simulink model "TST_EISGov_SelectParameter"  (R2016b)
settings: Solver=FixedStepDiscrete  StartTime=0.0  StopTime=simTime  FixedStep=sampleTime  RelTol=1e-3
values from neighbouring files (symbols this model uses):
  testCase = 1    [initTST_EISGov_SelectParameter_001.m]
libraries: simulink x26, UnitTest_Lib x24
(part 1 of 3)
settings Model: Creator=zhengjinyan  LastModifiedBy=zhengjinyan
settings DebuggingCC: SignalRangeChecking=error

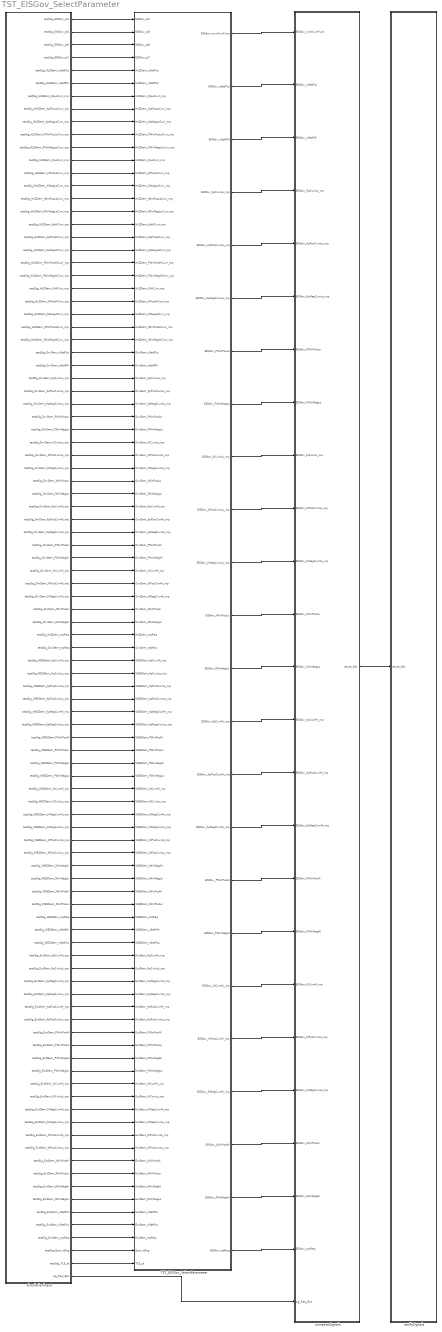
== system TST_EISGov_SelectParameter ==
  TST_EISGov_SelectParameter : Subsystem
  compareSignals : Subsystem
  simulationInput : Subsystem
  verifySignals : Subsystem
  wires:
  simulationInput/1(testSig_EISGov_st1) -> TST_EISGov_SelectParameter/1(EISGov_st1)
  simulationInput/2(testSig_EISGov_st3) -> TST_EISGov_SelectParameter/2(EISGov_st3)
  simulationInput/3(testSig_EISGov_st6) -> TST_EISGov_SelectParameter/3(EISGov_st6)
  simulationInput/4(testSig_EISGov_st7) -> TST_EISGov_SelectParameter/4(EISGov_st7)
  simulationInput/5(testSig_HLSDem_nSetPLo) -> TST_EISGov_SelectParameter/5(HLSDem_nSetPLo)
  simulationInput/6(testSig_HLSDem_nSetPHi) -> TST_EISGov_SelectParameter/6(HLSDem_nSetPHi)
  simulationInput/7(testSig_HLSDem_KpLoCurr_mp) -> TST_EISGov_SelectParameter/7(HLSDem_KpLoCurr_mp)
  simulationInput/8(testSig_HLSDem_KpPosLoCurr_mp) -> TST_EISGov_SelectParameter/8(HLSDem_KpPosLoCurr_mp)
  simulationInput/9(testSig_HLSDem_KpNegLoCurr_mp) -> TST_EISGov_SelectParameter/9(HLSDem_KpNegLoCurr_mp)
  simulationInput/10(testSig_HLSDem_PWinPosLoCurr_mp) -> TST_EISGov_SelectParameter/10(HLSDem_PWinPosLoCurr_mp)
  simulationInput/11(testSig_HLSDem_PWinNegLoCurr_mp) -> TST_EISGov_SelectParameter/11(HLSDem_PWinNegLoCurr_mp)
  simulationInput/12(testSig_HLSDem_KiLoCurr_mp) -> TST_EISGov_SelectParameter/12(HLSDem_KiLoCurr_mp)
  simulationInput/13(testSig_HLSDem_KiPosLoCurr_mp) -> TST_EISGov_SelectParameter/13(HLSDem_KiPosLoCurr_mp)
  simulationInput/14(testSig_HLSDem_KiNegLoCurr_mp) -> TST_EISGov_SelectParameter/14(HLSDem_KiNegLoCurr_mp)
  simulationInput/15(testSig_HLSDem_IWinPosLoCurr_mp) -> TST_EISGov_SelectParameter/15(HLSDem_IWinPosLoCurr_mp)
  simulationInput/16(testSig_HLSDem_IWinNegLoCurr_mp) -> TST_EISGov_SelectParameter/16(HLSDem_IWinNegLoCurr_mp)
  simulationInput/17(testSig_HLSDem_KpHiCurr_mp) -> TST_EISGov_SelectParameter/17(HLSDem_KpHiCurr_mp)
  simulationInput/18(testSig_HLSDem_KpPosHiCurr_mp) -> TST_EISGov_SelectParameter/18(HLSDem_KpPosHiCurr_mp)
  simulationInput/19(testSig_HLSDem_KpNegHiCurr_mp) -> TST_EISGov_SelectParameter/19(HLSDem_KpNegHiCurr_mp)
  simulationInput/20(testSig_HLSDem_PWinPosHiCurr_mp) -> TST_EISGov_SelectParameter/20(HLSDem_PWinPosHiCurr_mp)
  simulationInput/21(testSig_HLSDem_PWinNegHiCurr_mp) -> TST_EISGov_SelectParameter/21(HLSDem_PWinNegHiCurr_mp)
  simulationInput/22(testSig_HLSDem_KiHiCurr_mp) -> TST_EISGov_SelectParameter/22(HLSDem_KiHiCurr_mp)
  simulationInput/23(testSig_HLSDem_KiPosHiCurr_mp) -> TST_EISGov_SelectParameter/23(HLSDem_KiPosHiCurr_mp)
  simulationInput/24(testSig_HLSDem_KiNegHiCurr_mp) -> TST_EISGov_SelectParameter/24(HLSDem_KiNegHiCurr_mp)
  simulationInput/25(testSig_HLSDem_IWinPosHiCurr_mp) -> TST_EISGov_SelectParameter/25(HLSDem_IWinPosHiCurr_mp)
  simulationInput/26(testSig_HLSDem_IWinNegHiCurr_mp) -> TST_EISGov_SelectParameter/26(HLSDem_IWinNegHiCurr_mp)
  simulationInput/27(testSig_DrvDem_nSetPLo) -> TST_EISGov_SelectParameter/27(DrvDem_nSetPLo)
  simulationInput/28(testSig_DrvDem_nSetPHi) -> TST_EISGov_SelectParameter/28(DrvDem_nSetPHi)
  simulationInput/29(testSig_DrvDem_KpCurrLo_mp) -> TST_EISGov_SelectParameter/29(DrvDem_KpCurrLo_mp)
  simulationInput/30(testSig_DrvDem_KpPosCurrLo_mp) -> TST_EISGov_SelectParameter/30(DrvDem_KpPosCurrLo_mp)
  simulationInput/31(testSig_DrvDem_KpNegCurrLo_mp) -> TST_EISGov_SelectParameter/31(DrvDem_KpNegCurrLo_mp)
  simulationInput/32(testSig_DrvDem_PWinPosLo) -> TST_EISGov_SelectParameter/32(DrvDem_PWinPosLo)
  simulationInput/33(testSig_DrvDem_PWinNegLo) -> TST_EISGov_SelectParameter/33(DrvDem_PWinNegLo)
  simulationInput/34(testSig_DrvDem_KiCurrLo_mp) -> TST_EISGov_SelectParameter/34(DrvDem_KiCurrLo_mp)
  simulationInput/35(testSig_DrvDem_KiPosCurrLo_mp) -> TST_EISGov_SelectParameter/35(DrvDem_KiPosCurrLo_mp)
  simulationInput/36(testSig_DrvDem_KiNegCurrLo_mp) -> TST_EISGov_SelectParameter/36(DrvDem_KiNegCurrLo_mp)
  simulationInput/37(testSig_DrvDem_IWinPosLo) -> TST_EISGov_SelectParameter/37(DrvDem_IWinPosLo)
  simulationInput/38(testSig_DrvDem_IWinNegLo) -> TST_EISGov_SelectParameter/38(DrvDem_IWinNegLo)
  simulationInput/39(testSig_DrvDem_KpCurrHi_mp) -> TST_EISGov_SelectParameter/39(DrvDem_KpCurrHi_mp)
  simulationInput/40(testSig_DrvDem_KpPosCurrHi_mp) -> TST_EISGov_SelectParameter/40(DrvDem_KpPosCurrHi_mp)
  simulationInput/41(testSig_DrvDem_KpNegCurrHi_mp) -> TST_EISGov_SelectParameter/41(DrvDem_KpNegCurrHi_mp)
  simulationInput/42(testSig_DrvDem_PWinPosHi) -> TST_EISGov_SelectParameter/42(DrvDem_PWinPosHi)
  simulationInput/43(testSig_DrvDem_PWinNegHi) -> TST_EISGov_SelectParameter/43(DrvDem_PWinNegHi)
  simulationInput/44(testSig_DrvDem_KiCurrHi_mp) -> TST_EISGov_SelectParameter/44(DrvDem_KiCurrHi_mp)
  simulationInput/45(testSig_DrvDem_KiPosCurrHi_mp) -> TST_EISGov_SelectParameter/45(DrvDem_KiPosCurrHi_mp)
  simulationInput/46(testSig_DrvDem_KiNegCurrHi_mp) -> TST_EISGov_SelectParameter/46(DrvDem_KiNegCurrHi_mp)
  simulationInput/47(testSig_DrvDem_IWinPosHi) -> TST_EISGov_SelectParameter/47(DrvDem_IWinPosHi)
  simulationInput/48(testSig_DrvDem_IWinNegHi) -> TST_EISGov_SelectParameter/48(DrvDem_IWinNegHi)
  simulationInput/49(testSig_HLSDem_trqReq) -> TST_EISGov_SelectParameter/49(HLSDem_trqReq)
  simulationInput/50(testSig_DrvDem_trqReq) -> TST_EISGov_SelectParameter/50(DrvDem_trqReq)
  simulationInput/51(testSig_WESDem_KpCurrHi_mp) -> TST_EISGov_SelectParameter/51(WESDem_KpCurrHi_mp)
  simulationInput/52(testSig_WESDem_KpCurrLo_mp) -> TST_EISGov_SelectParameter/52(WESDem_KpCurrLo_mp)
  simulationInput/53(testSig_WESDem_KpPosCurrHi_mp) -> TST_EISGov_SelectParameter/53(WESDem_KpPosCurrHi_mp)
  simulationInput/54(testSig_WESDem_KpPosCurrLo_mp) -> TST_EISGov_SelectParameter/54(WESDem_KpPosCurrLo_mp)
  simulationInput/55(testSig_WESDem_KpNegCurrHi_mp) -> TST_EISGov_SelectParameter/55(WESDem_KpNegCurrHi_mp)
  simulationInput/56(testSig_WESDem_KpNegCurrLo_mp) -> TST_EISGov_SelectParameter/56(WESDem_KpNegCurrLo_mp)
  simulationInput/57(testSig_WESDem_PWinPosHi) -> TST_EISGov_SelectParameter/57(WESDem_PWinPosHi)
  simulationInput/58(testSig_WESDem_PWinPosLo) -> TST_EISGov_SelectParameter/58(WESDem_PWinPosLo)
  simulationInput/59(testSig_WESDem_PWinNegHi) -> TST_EISGov_SelectParameter/59(WESDem_PWinNegHi)
  simulationInput/60(testSig_WESDem_PWinNegLo) -> TST_EISGov_SelectParameter/60(WESDem_PWinNegLo)
  simulationInput/61(testSig_WESDem_KiCurrHi_mp) -> TST_EISGov_SelectParameter/61(WESDem_KiCurrHi_mp)
  simulationInput/62(testSig_WESDem_KiCurrLo_mp) -> TST_EISGov_SelectParameter/62(WESDem_KiCurrLo_mp)
  simulationInput/63(testSig_WESDem_KiNegCurrHi_mp) -> TST_EISGov_SelectParameter/63(WESDem_KiNegCurrHi_mp)
  simulationInput/64(testSig_WESDem_KiNegCurrLo_mp) -> TST_EISGov_SelectParameter/64(WESDem_KiNegCurrLo_mp)
  simulationInput/65(testSig_WESDem_KiPosCurrHi_mp) -> TST_EISGov_SelectParameter/65(WESDem_KiPosCurrHi_mp)
  simulationInput/66(testSig_WESDem_KiPosCurrLo_mp) -> TST_EISGov_SelectParameter/66(WESDem_KiPosCurrLo_mp)
  simulationInput/67(testSig_WESDem_IWinNegHi) -> TST_EISGov_SelectParameter/67(WESDem_IWinNegHi)
  simulationInput/68(testSig_WESDem_IWinNegLo) -> TST_EISGov_SelectParameter/68(WESDem_IWinNegLo)
  simulationInput/69(testSig_WESDem_IWinPosHi) -> TST_EISGov_SelectParameter/69(WESDem_IWinPosHi)
  simulationInput/70(testSig_WESDem_IWinPosLo) -> TST_EISGov_SelectParameter/70(WESDem_IWinPosLo)
  simulationInput/71(testSig_WESDem_trqReq) -> TST_EISGov_SelectParameter/71(WESDem_trqReq)
  simulationInput/72(testSig_WESDem_nSetPHi) -> TST_EISGov_SelectParameter/72(WESDem_nSetPHi)
  simulationInput/73(testSig_WESDem_nSetPLo) -> TST_EISGov_SelectParameter/73(WESDem_nSetPLo)
  simulationInput/74(testSig_ExtDem_KpCurrHi_mp) -> TST_EISGov_SelectParameter/74(ExtDem_KpCurrHi_mp)
  simulationInput/75(testSig_ExtDem_KpCurrLo_mp) -> TST_EISGov_SelectParameter/75(ExtDem_KpCurrLo_mp)
  simulationInput/76(testSig_ExtDem_KpNegCurrHi_mp) -> TST_EISGov_SelectParameter/76(ExtDem_KpNegCurrHi_mp)
  simulationInput/77(testSig_ExtDem_KpNegCurrLo_mp) -> TST_EISGov_SelectParameter/77(ExtDem_KpNegCurrLo_mp)
  simulationInput/78(testSig_ExtDem_KpPosCurrHi_mp) -> TST_EISGov_SelectParameter/78(ExtDem_KpPosCurrHi_mp)
  simulationInput/79(testSig_ExtDem_KpPosCurrLo_mp) -> TST_EISGov_SelectParameter/79(ExtDem_KpPosCurrLo_mp)
  simulationInput/80(testSig_ExtDem_PWinPosHi) -> TST_EISGov_SelectParameter/80(ExtDem_PWinPosHi)
  simulationInput/81(testSig_ExtDem_PWinPosLo) -> TST_EISGov_SelectParameter/81(ExtDem_PWinPosLo)
  simulationInput/82(testSig_ExtDem_PWinNegHi) -> TST_EISGov_SelectParameter/82(ExtDem_PWinNegHi)
  simulationInput/83(testSig_ExtDem_PWinNegLo) -> TST_EISGov_SelectParameter/83(ExtDem_PWinNegLo)
  simulationInput/84(testSig_ExtDem_KiCurrHi_mp) -> TST_EISGov_SelectParameter/84(ExtDem_KiCurrHi_mp)
  simulationInput/85(testSig_ExtDem_KiCurrLo_mp) -> TST_EISGov_SelectParameter/85(ExtDem_KiCurrLo_mp)
  simulationInput/86(testSig_ExtDem_KiNegCurrHi_mp) -> TST_EISGov_SelectParameter/86(ExtDem_KiNegCurrHi_mp)
  simulationInput/87(testSig_ExtDem_KiNegCurrLo_mp) -> TST_EISGov_SelectParameter/87(ExtDem_KiNegCurrLo_mp)
  simulationInput/88(testSig_ExtDem_KiPosCurrHi_mp) -> TST_EISGov_SelectParameter/88(ExtDem_KiPosCurrHi_mp)
  simulationInput/89(testSig_ExtDem_KiPosCurrLo_mp) -> TST_EISGov_SelectParameter/89(ExtDem_KiPosCurrLo_mp)
  simulationInput/90(testSig_ExtDem_IWinPosHi) -> TST_EISGov_SelectParameter/90(ExtDem_IWinPosHi)
  simulationInput/91(testSig_ExtDem_IWinPosLo) -> TST_EISGov_SelectParameter/91(ExtDem_IWinPosLo)
  simulationInput/92(testSig_ExtDem_IWinNegHi) -> TST_EISGov_SelectParameter/92(ExtDem_IWinNegHi)
  simulationInput/93(testSig_ExtDem_IWinNegLo) -> TST_EISGov_SelectParameter/93(ExtDem_IWinNegLo)
  simulationInput/94(testSig_ExtDem_nSetPHi) -> TST_EISGov_SelectParameter/94(ExtDem_nSetPHi)
  simulationInput/95(testSig_ExtDem_nSetPLo) -> TST_EISGov_SelectParameter/95(ExtDem_nSetPLo)
  simulationInput/96(testSig_ExtDem_trqReq) -> TST_EISGov_SelectParameter/96(ExtDem_trqReq)
  simulationInput/97(testSig_Epm_nEng) -> TST_EISGov_SelectParameter/97(Epm_nEng)
  simulationInput/98(testSig_T15_st) -> TST_EISGov_SelectParameter/98(T15_st)
  TST_EISGov_SelectParameter/1(EISGov_numCurrFunc) -> compareSignals/1(EISGov_numCurrFunc)
  TST_EISGov_SelectParameter/2(EISGov_nSetPLo) -> compareSignals/2(EISGov_nSetPLo)
  TST_EISGov_SelectParameter/3(EISGov_nSetPHi) -> compareSignals/3(EISGov_nSetPHi)
  TST_EISGov_SelectParameter/4(EISGov_KpCurrLo_mp) -> compareSignals/4(EISGov_KpCurrLo_mp)
  TST_EISGov_SelectParameter/5(EISGov_KpPosCurrLo_mp) -> compareSignals/5(EISGov_KpPosCurrLo_mp)
  TST_EISGov_SelectParameter/6(EISGov_KpNegCurrLo_mp) -> compareSignals/6(EISGov_KpNegCurrLo_mp)
  TST_EISGov_SelectParameter/7(EISGov_PWinPosLo) -> compareSignals/7(EISGov_PWinPosLo)
  TST_EISGov_SelectParameter/8(EISGov_PWinNegLo) -> compareSignals/8(EISGov_PWinNegLo)
  TST_EISGov_SelectParameter/9(EISGov_KiCurrLo_mp) -> compareSignals/9(EISGov_KiCurrLo_mp)
  TST_EISGov_SelectParameter/10(EISGov_KiPosCurrLo_mp) -> compareSignals/10(EISGov_KiPosCurrLo_mp)
  TST_EISGov_SelectParameter/11(EISGov_KiNegCurrLo_mp) -> compareSignals/11(EISGov_KiNegCurrLo_mp)
  TST_EISGov_SelectParameter/12(EISGov_IWinPosLo) -> compareSignals/12(EISGov_IWinPosLo)
  TST_EISGov_SelectParameter/13(EISGov_IWinNegLo) -> compareSignals/13(EISGov_IWinNegLo)
  TST_EISGov_SelectParameter/14(EISGov_KpCurrHi_mp) -> compareSignals/14(EISGov_KpCurrHi_mp)
  TST_EISGov_SelectParameter/15(EISGov_KpPosCurrHi_mp) -> compareSignals/15(EISGov_KpPosCurrHi_mp)
  TST_EISGov_SelectParameter/16(EISGov_KpNegCurrHi_mp) -> compareSignals/16(EISGov_KpNegCurrHi_mp)
  TST_EISGov_SelectParameter/17(EISGov_PWinPosHi) -> compareSignals/17(EISGov_PWinPosHi)
  TST_EISGov_SelectParameter/18(EISGov_PWinNegHi) -> compareSignals/18(EISGov_PWinNegHi)
  TST_EISGov_SelectParameter/19(EISGov_KiCurrHi_mp) -> compareSignals/19(EISGov_KiCurrHi_mp)
  TST_EISGov_SelectParameter/20(EISGov_KiPosCurrHi_mp) -> compareSignals/20(EISGov_KiPosCurrHi_mp)
  TST_EISGov_SelectParameter/21(EISGov_KiNegCurrHi_mp) -> compareSignals/21(EISGov_KiNegCurrHi_mp)
  TST_EISGov_SelectParameter/22(EISGov_IWinPosHi) -> compareSignals/22(EISGov_IWinPosHi)
  TST_EISGov_SelectParameter/23(EISGov_IWinNegHi) -> compareSignals/23(EISGov_IWinNegHi)
  TST_EISGov_SelectParameter/24(EISGov_trqReq) -> compareSignals/24(EISGov_trqReq)
  simulationInput/99(sig_Req_Bus) -> compareSignals/25(sig_Req_Bus)
  compareSignals/1(result_001) -> verifySignals/1(result_001)

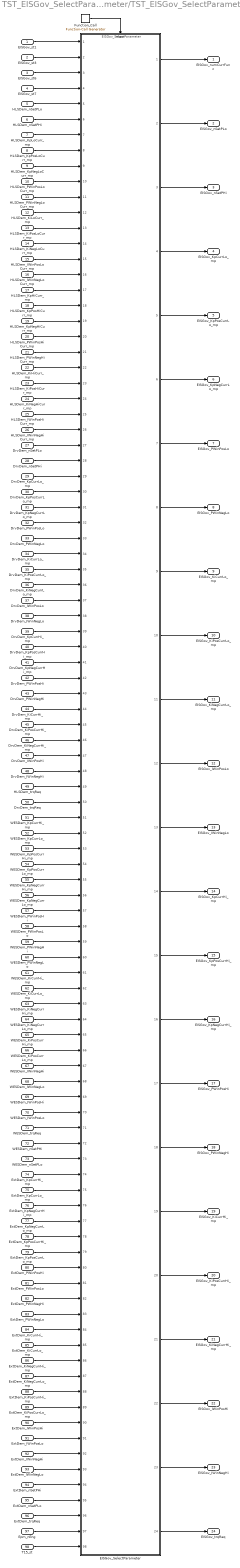
== system TST_EISGov_SelectParameter/TST_EISGov_SelectParameter ==
  EISGov_st1 : Inport
  EISGov_st3 : Inport  Port=2
  EISGov_st6 : Inport  Port=3
  EISGov_st7 : Inport  Port=4
  HLSDem_nSetPLo : Inport  Port=5
  HLSDem_nSetPHi : Inport  Port=6
  HLSDem_KpLoCurr_mp : Inport  Port=7
  HLSDem_KpPosLoCurr_mp : Inport  Port=8
  HLSDem_KpNegLoCurr_mp : Inport  Port=9
  HLSDem_PWinPosLoCurr_mp : Inport  Port=10
  HLSDem_PWinNegLoCurr_mp : Inport  Port=11
  HLSDem_KiLoCurr_mp : Inport  Port=12
  HLSDem_KiPosLoCurr_mp : Inport  Port=13
  HLSDem_KiNegLoCurr_mp : Inport  Port=14
  HLSDem_IWinPosLoCurr_mp : Inport  Port=15
  HLSDem_IWinNegLoCurr_mp : Inport  Port=16
  HLSDem_KpHiCurr_mp : Inport  Port=17
  HLSDem_KpPosHiCurr_mp : Inport  Port=18
  HLSDem_KpNegHiCurr_mp : Inport  Port=19
  HLSDem_PWinPosHiCurr_mp : Inport  Port=20
  HLSDem_PWinNegHiCurr_mp : Inport  Port=21
  HLSDem_KiHiCurr_mp : Inport  Port=22
  HLSDem_KiPosHiCurr_mp : Inport  Port=23
  HLSDem_KiNegHiCurr_mp : Inport  Port=24
  HLSDem_IWinPosHiCurr_mp : Inport  Port=25
  HLSDem_IWinNegHiCurr_mp : Inport  Port=26
  DrvDem_nSetPLo : Inport  Port=27
  DrvDem_nSetPHi : Inport  Port=28
  DrvDem_KpCurrLo_mp : Inport  Port=29
  DrvDem_KpPosCurrLo_mp : Inport  Port=30
  DrvDem_KpNegCurrLo_mp : Inport  Port=31
  DrvDem_PWinPosLo : Inport  Port=32
  DrvDem_PWinNegLo : Inport  Port=33
  DrvDem_KiCurrLo_mp : Inport  Port=34
  DrvDem_KiPosCurrLo_mp : Inport  Port=35
  DrvDem_KiNegCurrLo_mp : Inport  Port=36
  DrvDem_IWinPosLo : Inport  Port=37
  DrvDem_IWinNegLo : Inport  Port=38
  DrvDem_KpCurrHi_mp : Inport  Port=39
  DrvDem_KpPosCurrHi_mp : Inport  Port=40
  DrvDem_KpNegCurrHi_mp : Inport  Port=41
  DrvDem_PWinPosHi : Inport  Port=42
  DrvDem_PWinNegHi : Inport  Port=43
  DrvDem_KiCurrHi_mp : Inport  Port=44
  DrvDem_KiPosCurrHi_mp : Inport  Port=45
  DrvDem_KiNegCurrHi_mp : Inport  Port=46
  DrvDem_IWinPosHi : Inport  Port=47
  DrvDem_IWinNegHi : Inport  Port=48
  HLSDem_trqReq : Inport  Port=49
  DrvDem_trqReq : Inport  Port=50
  WESDem_KpCurrHi_mp : Inport  Port=51
  WESDem_KpCurrLo_mp : Inport  Port=52
  WESDem_KpPosCurrHi_mp : Inport  Port=53
  WESDem_KpPosCurrLo_mp : Inport  Port=54
  WESDem_KpNegCurrHi_mp : Inport  Port=55
  WESDem_KpNegCurrLo_mp : Inport  Port=56
  WESDem_PWinPosHi : Inport  Port=57
  WESDem_PWinPosLo : Inport  Port=58
  WESDem_PWinNegHi : Inport  Port=59
  WESDem_PWinNegLo : Inport  Port=60
  WESDem_KiCurrHi_mp : Inport  Port=61
  WESDem_KiCurrLo_mp : Inport  Port=62
  WESDem_KiNegCurrHi_mp : Inport  Port=63
  WESDem_KiNegCurrLo_mp : Inport  Port=64
  WESDem_KiPosCurrHi_mp : Inport  Port=65
  WESDem_KiPosCurrLo_mp : Inport  Port=66
  WESDem_IWinNegHi : Inport  Port=67
  WESDem_IWinNegLo : Inport  Port=68
  WESDem_IWinPosHi : Inport  Port=69
  WESDem_IWinPosLo : Inport  Port=70
  WESDem_trqReq : Inport  Port=71
  WESDem_nSetPHi : Inport  Port=72
  WESDem_nSetPLo : Inport  Port=73
  ExtDem_KpCurrHi_mp : Inport  Port=74
  ExtDem_KpCurrLo_mp : Inport  Port=75
  ExtDem_KpNegCurrHi_mp : Inport  Port=76
  ExtDem_KpNegCurrLo_mp : Inport  Port=77
  ExtDem_KpPosCurrHi_mp : Inport  Port=78
  ExtDem_KpPosCurrLo_mp : Inport  Port=79
  ExtDem_PWinPosHi : Inport  Port=80
  ExtDem_PWinPosLo : Inport  Port=81
  ExtDem_PWinNegHi : Inport  Port=82
  ExtDem_PWinNegLo : Inport  Port=83
  ExtDem_KiCurrHi_mp : Inport  Port=84
  ExtDem_KiCurrLo_mp : Inport  Port=85
  ExtDem_KiNegCurrHi_mp : Inport  Port=86
  ExtDem_KiNegCurrLo_mp : Inport  Port=87
  ExtDem_KiPosCurrHi_mp : Inport  Port=88
  ExtDem_KiPosCurrLo_mp : Inport  Port=89
  ExtDem_IWinPosHi : Inport  Port=90
  ExtDem_IWinPosLo : Inport  Port=91
  ExtDem_IWinNegHi : Inport  Port=92
  ExtDem_IWinNegLo : Inport  Port=93
  ExtDem_nSetPHi : Inport  Port=94
  ExtDem_nSetPLo : Inport  Port=95
  ExtDem_trqReq : Inport  Port=96
  Epm_nEng : Inport  Port=97
  T15_st : Inport  Port=98
  EISGov_SelectParameter : ModelReference  ModelNameDialog=EISGov_SelectParameter  SimulationMode=Normal  ModelReferenceVersion=1.180  TriggerPortName=function  TriggerPortTriggerType=function-call  TriggerPortStatesWhenEnabling=held
  Function_Call : simulink/Ports & Subsystems/Function-Call Generator  sample_time=sampleTime  numberOfIterations=1
  EISGov_numCurrFunc : Outport
  EISGov_nSetPLo : Outport  Port=2
  EISGov_nSetPHi : Outport  Port=3
  EISGov_KpCurrLo_mp : Outport  Port=4
  EISGov_KpPosCurrLo_mp : Outport  Port=5
  EISGov_KpNegCurrLo_mp : Outport  Port=6
  EISGov_PWinPosLo : Outport  Port=7
  EISGov_PWinNegLo : Outport  Port=8
  EISGov_KiCurrLo_mp : Outport  Port=9
  EISGov_KiPosCurrLo_mp : Outport  Port=10
  EISGov_KiNegCurrLo_mp : Outport  Port=11
  EISGov_IWinPosLo : Outport  Port=12
  EISGov_IWinNegLo : Outport  Port=13
  EISGov_KpCurrHi_mp : Outport  Port=14
  EISGov_KpPosCurrHi_mp : Outport  Port=15
  EISGov_KpNegCurrHi_mp : Outport  Port=16
  EISGov_PWinPosHi : Outport  Port=17
  EISGov_PWinNegHi : Outport  Port=18
  EISGov_KiCurrHi_mp : Outport  Port=19
  EISGov_KiPosCurrHi_mp : Outport  Port=20
  EISGov_KiNegCurrHi_mp : Outport  Port=21
  EISGov_IWinPosHi : Outport  Port=22
  EISGov_IWinNegHi : Outport  Port=23
  EISGov_trqReq : Outport  Port=24
  wires:
  Function_Call/1 -> EISGov_SelectParameter/Trigger
  EISGov_st1/1 -> EISGov_SelectParameter/1
  EISGov_st3/1 -> EISGov_SelectParameter/2
  EISGov_st6/1 -> EISGov_SelectParameter/3
  EISGov_st7/1 -> EISGov_SelectParameter/4
  HLSDem_nSetPLo/1 -> EISGov_SelectParameter/5
  HLSDem_nSetPHi/1 -> EISGov_SelectParameter/6
  HLSDem_KpLoCurr_mp/1 -> EISGov_SelectParameter/7
  HLSDem_KpPosLoCurr_mp/1 -> EISGov_SelectParameter/8
  HLSDem_KpNegLoCurr_mp/1 -> EISGov_SelectParameter/9
  HLSDem_PWinPosLoCurr_mp/1 -> EISGov_SelectParameter/10
  HLSDem_PWinNegLoCurr_mp/1 -> EISGov_SelectParameter/11
  HLSDem_KiLoCurr_mp/1 -> EISGov_SelectParameter/12
  HLSDem_KiPosLoCurr_mp/1 -> EISGov_SelectParameter/13
  HLSDem_KiNegLoCurr_mp/1 -> EISGov_SelectParameter/14
  HLSDem_IWinPosLoCurr_mp/1 -> EISGov_SelectParameter/15
  HLSDem_IWinNegLoCurr_mp/1 -> EISGov_SelectParameter/16
  HLSDem_KpHiCurr_mp/1 -> EISGov_SelectParameter/17
  HLSDem_KpPosHiCurr_mp/1 -> EISGov_SelectParameter/18
  HLSDem_KpNegHiCurr_mp/1 -> EISGov_SelectParameter/19
  HLSDem_PWinPosHiCurr_mp/1 -> EISGov_SelectParameter/20
  HLSDem_PWinNegHiCurr_mp/1 -> EISGov_SelectParameter/21
  HLSDem_KiHiCurr_mp/1 -> EISGov_SelectParameter/22
  HLSDem_KiPosHiCurr_mp/1 -> EISGov_SelectParameter/23
  HLSDem_KiNegHiCurr_mp/1 -> EISGov_SelectParameter/24
  HLSDem_IWinPosHiCurr_mp/1 -> EISGov_SelectParameter/25
  HLSDem_IWinNegHiCurr_mp/1 -> EISGov_SelectParameter/26
  DrvDem_nSetPLo/1 -> EISGov_SelectParameter/27
  DrvDem_nSetPHi/1 -> EISGov_SelectParameter/28
  DrvDem_KpCurrLo_mp/1 -> EISGov_SelectParameter/29
  DrvDem_KpPosCurrLo_mp/1 -> EISGov_SelectParameter/30
  DrvDem_KpNegCurrLo_mp/1 -> EISGov_SelectParameter/31
  DrvDem_PWinPosLo/1 -> EISGov_SelectParameter/32
  DrvDem_PWinNegLo/1 -> EISGov_SelectParameter/33
  DrvDem_KiCurrLo_mp/1 -> EISGov_SelectParameter/34
  DrvDem_KiPosCurrLo_mp/1 -> EISGov_SelectParameter/35
  DrvDem_KiNegCurrLo_mp/1 -> EISGov_SelectParameter/36
  DrvDem_IWinPosLo/1 -> EISGov_SelectParameter/37
  DrvDem_IWinNegLo/1 -> EISGov_SelectParameter/38
  DrvDem_KpCurrHi_mp/1 -> EISGov_SelectParameter/39
  DrvDem_KpPosCurrHi_mp/1 -> EISGov_SelectParameter/40
  DrvDem_KpNegCurrHi_mp/1 -> EISGov_SelectParameter/41
  DrvDem_PWinPosHi/1 -> EISGov_SelectParameter/42
  DrvDem_PWinNegHi/1 -> EISGov_SelectParameter/43
  DrvDem_KiCurrHi_mp/1 -> EISGov_SelectParameter/44
  DrvDem_KiPosCurrHi_mp/1 -> EISGov_SelectParameter/45
  DrvDem_KiNegCurrHi_mp/1 -> EISGov_SelectParameter/46
  DrvDem_IWinPosHi/1 -> EISGov_SelectParameter/47
  DrvDem_IWinNegHi/1 -> EISGov_SelectParameter/48
  HLSDem_trqReq/1 -> EISGov_SelectParameter/49
  DrvDem_trqReq/1 -> EISGov_SelectParameter/50
  WESDem_KpCurrHi_mp/1 -> EISGov_SelectParameter/51
  WESDem_KpCurrLo_mp/1 -> EISGov_SelectParameter/52
  WESDem_KpPosCurrHi_mp/1 -> EISGov_SelectParameter/53
  WESDem_KpPosCurrLo_mp/1 -> EISGov_SelectParameter/54
  WESDem_KpNegCurrHi_mp/1 -> EISGov_SelectParameter/55
  WESDem_KpNegCurrLo_mp/1 -> EISGov_SelectParameter/56
  WESDem_PWinPosHi/1 -> EISGov_SelectParameter/57
  WESDem_PWinPosLo/1 -> EISGov_SelectParameter/58
  WESDem_PWinNegHi/1 -> EISGov_SelectParameter/59
  WESDem_PWinNegLo/1 -> EISGov_SelectParameter/60
  WESDem_KiCurrHi_mp/1 -> EISGov_SelectParameter/61
  WESDem_KiCurrLo_mp/1 -> EISGov_SelectParameter/62
  WESDem_KiNegCurrHi_mp/1 -> EISGov_SelectParameter/63
  WESDem_KiNegCurrLo_mp/1 -> EISGov_SelectParameter/64
  WESDem_KiPosCurrHi_mp/1 -> EISGov_SelectParameter/65
  WESDem_KiPosCurrLo_mp/1 -> EISGov_SelectParameter/66
  WESDem_IWinNegHi/1 -> EISGov_SelectParameter/67
  WESDem_IWinNegLo/1 -> EISGov_SelectParameter/68
  WESDem_IWinPosHi/1 -> EISGov_SelectParameter/69
  WESDem_IWinPosLo/1 -> EISGov_SelectParameter/70
  WESDem_trqReq/1 -> EISGov_SelectParameter/71
  WESDem_nSetPHi/1 -> EISGov_SelectParameter/72
  WESDem_nSetPLo/1 -> EISGov_SelectParameter/73
  ExtDem_KpCurrHi_mp/1 -> EISGov_SelectParameter/74
  ExtDem_KpCurrLo_mp/1 -> EISGov_SelectParameter/75
  ExtDem_KpNegCurrHi_mp/1 -> EISGov_SelectParameter/76
  ExtDem_KpNegCurrLo_mp/1 -> EISGov_SelectParameter/77
  ExtDem_KpPosCurrHi_mp/1 -> EISGov_SelectParameter/78
  ExtDem_KpPosCurrLo_mp/1 -> EISGov_SelectParameter/79
  ExtDem_PWinPosHi/1 -> EISGov_SelectParameter/80
  ExtDem_PWinPosLo/1 -> EISGov_SelectParameter/81
  ExtDem_PWinNegHi/1 -> EISGov_SelectParameter/82
  ExtDem_PWinNegLo/1 -> EISGov_SelectParameter/83
  ExtDem_KiCurrHi_mp/1 -> EISGov_SelectParameter/84
  ExtDem_KiCurrLo_mp/1 -> EISGov_SelectParameter/85
  ExtDem_KiNegCurrHi_mp/1 -> EISGov_SelectParameter/86
  ExtDem_KiNegCurrLo_mp/1 -> EISGov_SelectParameter/87
  ExtDem_KiPosCurrHi_mp/1 -> EISGov_SelectParameter/88
  ExtDem_KiPosCurrLo_mp/1 -> EISGov_SelectParameter/89
  ExtDem_IWinPosHi/1 -> EISGov_SelectParameter/90
  ExtDem_IWinPosLo/1 -> EISGov_SelectParameter/91
  ExtDem_IWinNegHi/1 -> EISGov_SelectParameter/92
  ExtDem_IWinNegLo/1 -> EISGov_SelectParameter/93
  ExtDem_nSetPHi/1 -> EISGov_SelectParameter/94
  ExtDem_nSetPLo/1 -> EISGov_SelectParameter/95
  ExtDem_trqReq/1 -> EISGov_SelectParameter/96
  Epm_nEng/1 -> EISGov_SelectParameter/97
  T15_st/1 -> EISGov_SelectParameter/98
  EISGov_SelectParameter/1 -> EISGov_numCurrFunc/1
  EISGov_SelectParameter/2 -> EISGov_nSetPLo/1
  EISGov_SelectParameter/3 -> EISGov_nSetPHi/1
  EISGov_SelectParameter/4 -> EISGov_KpCurrLo_mp/1
  EISGov_SelectParameter/5 -> EISGov_KpPosCurrLo_mp/1
  EISGov_SelectParameter/6 -> EISGov_KpNegCurrLo_mp/1
  EISGov_SelectParameter/7 -> EISGov_PWinPosLo/1
  EISGov_SelectParameter/8 -> EISGov_PWinNegLo/1
  EISGov_SelectParameter/9 -> EISGov_KiCurrLo_mp/1
  EISGov_SelectParameter/10 -> EISGov_KiPosCurrLo_mp/1
  EISGov_SelectParameter/11 -> EISGov_KiNegCurrLo_mp/1
  EISGov_SelectParameter/12 -> EISGov_IWinPosLo/1
  EISGov_SelectParameter/13 -> EISGov_IWinNegLo/1
  EISGov_SelectParameter/14 -> EISGov_KpCurrHi_mp/1
  EISGov_SelectParameter/15 -> EISGov_KpPosCurrHi_mp/1
  EISGov_SelectParameter/16 -> EISGov_KpNegCurrHi_mp/1
  EISGov_SelectParameter/17 -> EISGov_PWinPosHi/1
  EISGov_SelectParameter/18 -> EISGov_PWinNegHi/1
  EISGov_SelectParameter/19 -> EISGov_KiCurrHi_mp/1
  EISGov_SelectParameter/20 -> EISGov_KiPosCurrHi_mp/1
  EISGov_SelectParameter/21 -> EISGov_KiNegCurrHi_mp/1
  EISGov_SelectParameter/22 -> EISGov_IWinPosHi/1
  EISGov_SelectParameter/23 -> EISGov_IWinNegHi/1
  EISGov_SelectParameter/24 -> EISGov_trqReq/1

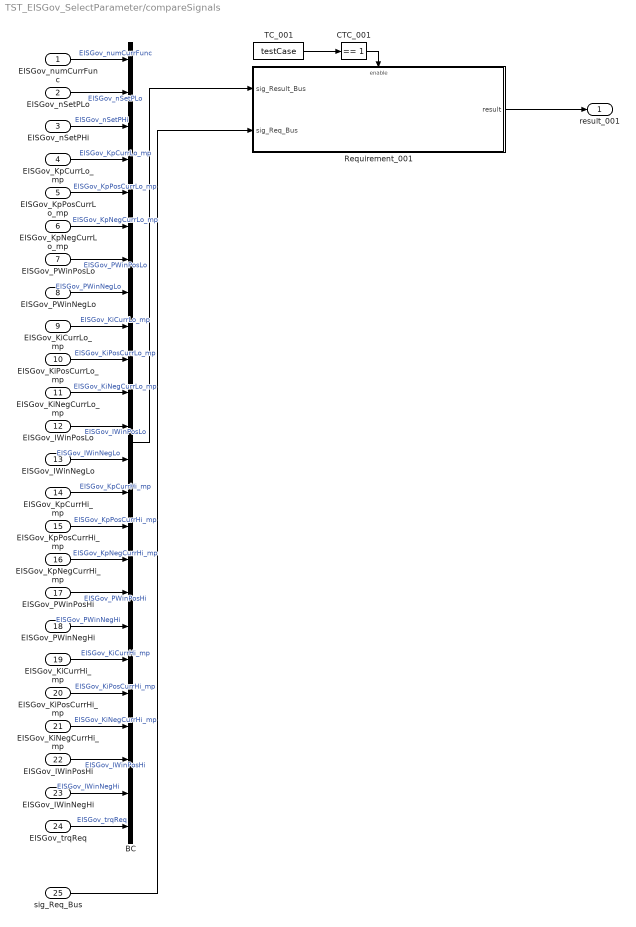
== system TST_EISGov_SelectParameter/compareSignals ==
  EISGov_numCurrFunc : Inport
  EISGov_nSetPLo : Inport  Port=2
  EISGov_nSetPHi : Inport  Port=3
  EISGov_KpCurrLo_mp : Inport  Port=4
  EISGov_KpPosCurrLo_mp : Inport  Port=5
  EISGov_KpNegCurrLo_mp : Inport  Port=6
  EISGov_PWinPosLo : Inport  Port=7
  EISGov_PWinNegLo : Inport  Port=8
  EISGov_KiCurrLo_mp : Inport  Port=9
  EISGov_KiPosCurrLo_mp : Inport  Port=10
  EISGov_KiNegCurrLo_mp : Inport  Port=11
  EISGov_IWinPosLo : Inport  Port=12
  EISGov_IWinNegLo : Inport  Port=13
  EISGov_KpCurrHi_mp : Inport  Port=14
  EISGov_KpPosCurrHi_mp : Inport  Port=15
  EISGov_KpNegCurrHi_mp : Inport  Port=16
  EISGov_PWinPosHi : Inport  Port=17
  EISGov_PWinNegHi : Inport  Port=18
  EISGov_KiCurrHi_mp : Inport  Port=19
  EISGov_KiPosCurrHi_mp : Inport  Port=20
  EISGov_KiNegCurrHi_mp : Inport  Port=21
  EISGov_IWinPosHi : Inport  Port=22
  EISGov_IWinNegHi : Inport  Port=23
  EISGov_trqReq : Inport  Port=24
  sig_Req_Bus : Inport  Port=25
  BC : BusCreator  Inputs=24
  CTC_001 : simulink/Logic and Bit Operations/Compare To Constant  relop===  const=1  OutDataTypeStr=boolean
  Requirement_001 : Subsystem
  TC_001 : Constant  Value=testCase
  result_001 : Outport
  wires:
  EISGov_numCurrFunc/1 -> BC/1  "EISGov_numCurrFunc"
  EISGov_nSetPLo/1 -> BC/2  "EISGov_nSetPLo"
  EISGov_nSetPHi/1 -> BC/3  "EISGov_nSetPHi"
  EISGov_KpCurrLo_mp/1 -> BC/4  "EISGov_KpCurrLo_mp"
  EISGov_KpPosCurrLo_mp/1 -> BC/5  "EISGov_KpPosCurrLo_mp"
  EISGov_KpNegCurrLo_mp/1 -> BC/6  "EISGov_KpNegCurrLo_mp"
  EISGov_PWinPosLo/1 -> BC/7  "EISGov_PWinPosLo"
  EISGov_PWinNegLo/1 -> BC/8  "EISGov_PWinNegLo"
  EISGov_KiCurrLo_mp/1 -> BC/9  "EISGov_KiCurrLo_mp"
  EISGov_KiPosCurrLo_mp/1 -> BC/10  "EISGov_KiPosCurrLo_mp"
  EISGov_KiNegCurrLo_mp/1 -> BC/11  "EISGov_KiNegCurrLo_mp"
  EISGov_IWinPosLo/1 -> BC/12  "EISGov_IWinPosLo"
  EISGov_IWinNegLo/1 -> BC/13  "EISGov_IWinNegLo"
  EISGov_KpCurrHi_mp/1 -> BC/14  "EISGov_KpCurrHi_mp"
  EISGov_KpPosCurrHi_mp/1 -> BC/15  "EISGov_KpPosCurrHi_mp"
  EISGov_KpNegCurrHi_mp/1 -> BC/16  "EISGov_KpNegCurrHi_mp"
  EISGov_PWinPosHi/1 -> BC/17  "EISGov_PWinPosHi"
  EISGov_PWinNegHi/1 -> BC/18  "EISGov_PWinNegHi"
  EISGov_KiCurrHi_mp/1 -> BC/19  "EISGov_KiCurrHi_mp"
  EISGov_KiPosCurrHi_mp/1 -> BC/20  "EISGov_KiPosCurrHi_mp"
  EISGov_KiNegCurrHi_mp/1 -> BC/21  "EISGov_KiNegCurrHi_mp"
  EISGov_IWinPosHi/1 -> BC/22  "EISGov_IWinPosHi"
  EISGov_IWinNegHi/1 -> BC/23  "EISGov_IWinNegHi"
  EISGov_trqReq/1 -> BC/24  "EISGov_trqReq"
  TC_001/1 -> CTC_001/1
  CTC_001/1 -> Requirement_001/Enable
  sig_Req_Bus/1 -> Requirement_001/2(sig_Req_Bus)
  BC/1 -> Requirement_001/1(sig_Result_Bus)
  Requirement_001/1(result) -> result_001/1

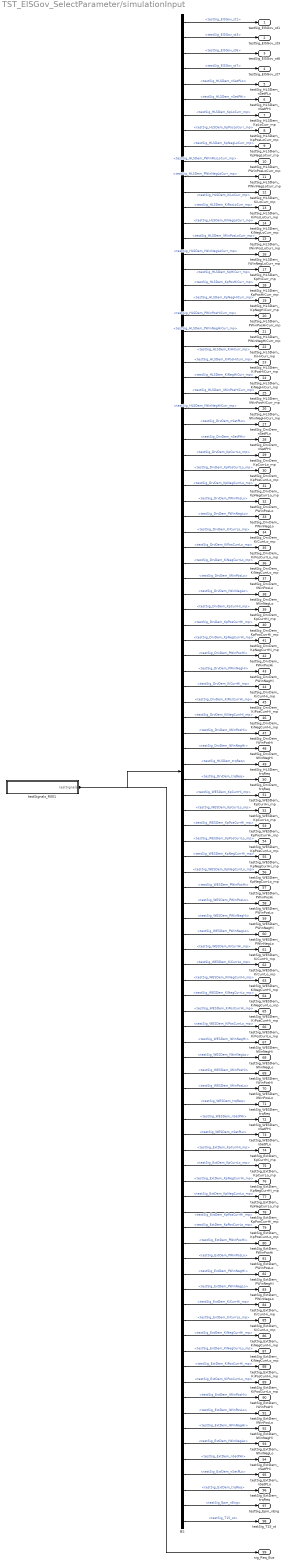
== system TST_EISGov_SelectParameter/simulationInput ==
  BS : BusSelector  OutputSignals=testSig_EISGov_st1,testSig_EISGov_st3,testSig_EISGov_st6,testSig_EISGov_st7,testSig_HLSDem_nSetPLo,testSig_HLSDem_nSetPHi,testSig_HLSDem_KpLoCurr_mp,testSig_HLSDem_KpPosLoCurr_mp,testSig_HLSDem_KpNegLoCurr_mp,testSig_HLSDem_PWinPosLoCurr_mp,testSig_HLSDem_PWinNegLoCurr_mp,testSig_HLSDem_KiLoCurr_mp,testSig_HLSDem_KiPosLoCurr_mp,testSig_HLSDem_KiNegLoCurr_mp,testSig_HLSDem_IWinPosLoCurr_mp,testSig_HLSDem_IWinNegLoCurr_mp,testSig_HLSDem_KpHiCurr_mp,testSig_HLSDem_KpPosHiCurr_mp,testSig_HLSDem_KpNegHiCurr_mp,testSig_HLSDem_PWinPosHiCurr_mp,testSig_HLSDem_PWinNegHiCurr_mp,testSig_HLSDem_KiHiCurr_mp,testSig_HLSDem_KiPosHiCurr_mp,testSig_HLSDem_KiNegHiCurr_mp,testSig_HLSDem_IWinPosHiCurr_mp,testSig_HLSDem_IWinNegHiCurr_mp,testSig_DrvDem_nSetPLo,testSig_DrvDem_nSetPHi,testSig_DrvDem_KpCurrLo_mp,testSig_DrvDem_KpPosCurrLo_mp,testSig_DrvDem_KpNegCurrLo_mp,testSig_DrvDem_PWinPosLo,testSig_DrvDem_PWinNegLo,testSig_DrvDem_KiCurrLo_mp,testSig_DrvDem_KiPosCurrLo_mp,testSig_DrvDem_KiNegCurrLo_mp,testSig_DrvDem_IWinPosLo,testSig_DrvDem_IWinNegLo,testSig_DrvDem_KpCurrHi_mp,testSig_DrvDem_KpPosCurrHi_mp,testSig_DrvDem_KpNegCurrHi_mp,testSig_DrvDem_PWinPosHi,testSig_DrvDem_PWinNegHi,testSig_DrvDem_KiCurrHi_mp,testSig_DrvDem_KiPosCurrHi_mp,testSig_DrvDem_KiNegCurrHi_mp,testSig_DrvDem_IWinPosHi,testSig_DrvDem_IWinNegHi,testSig_HLSDem_trqReq,testSig_DrvDem_trqReq,testSig_WESDem_KpCurrHi_mp,testSig_WESDem_KpCurrLo_mp,testSig_WESDem_KpPosCurrHi_mp,testSig_WESDem_KpPosCurrLo_mp,testSig_WESDem_KpNegCurrHi_mp,testSig_WESDem_KpNegCurrLo_mp,testSig_WESDem_PWinPosHi,testSig_WESDem_PWinPosLo,testSig_WESDem_PWinNegHi,testSig_WESDem_PWinNegLo,testSig_WESDem_KiCurrHi_mp,testSig_WESDem_KiCurrLo_mp,testSig_WESDem_KiNegCurrHi_mp,testSig_WESDem_KiNegCurrLo_mp,testSig_WESDem_KiPosCurrHi_mp,testSig_WESDem_KiPosCurrLo_mp,testSig_WESDem_IWinNegHi,testSig_WESDem_IWinNegLo,testSig_WESDem_IWinPosHi,testSig_WESDem_IWinPosLo,testSig_WESDem_trqReq,testSig_WESDem_nSetPHi,testSig_WESDem_nSetPLo,testSig_ExtDem_KpCurrHi_mp,testSig_ExtDem_KpCurrLo_mp,testSig_ExtDem_KpNegCurrHi_mp,testSig_ExtDem_KpNegCurrLo_mp,testSig_ExtDem_KpPosCurrHi_mp,testSig_ExtDem_KpPosCurrLo_mp,testSig_ExtDem_PWinPosHi,testSig_ExtDem_PWinPosLo,testSig_ExtDem_PWinNegHi,testSig_ExtDem_PWinNegLo,testSig_ExtDem_KiCurrHi_mp,testSig_ExtDem_KiCurrLo_mp,testSig_ExtDem_KiNegCurrHi_mp,testSig_ExtDem_KiNegCurrLo_mp,testSig_ExtDem_KiPosCurrHi_mp,testSig_ExtDem_KiPosCurrLo_mp,testSig_ExtDem_IWinPosHi,testSig_ExtDem_IWinPosLo,testSig_ExtDem_IWinNegHi,testSig_ExtDem_IWinNegLo,testSig_ExtDem_nSetPHi,testSig_ExtDem_nSetPLo,testSig_ExtDem_trqReq,testSig_Epm_nEng,testSig_T15_st
  testSignals_R001 : Subsystem
  testSig_EISGov_st1 : Outport
  testSig_EISGov_st3 : Outport  Port=2
  testSig_EISGov_st6 : Outport  Port=3
  testSig_EISGov_st7 : Outport  Port=4
  testSig_HLSDem_nSetPLo : Outport  Port=5
  testSig_HLSDem_nSetPHi : Outport  Port=6
  testSig_HLSDem_KpLoCurr_mp : Outport  Port=7
  testSig_HLSDem_KpPosLoCurr_mp : Outport  Port=8
  testSig_HLSDem_KpNegLoCurr_mp : Outport  Port=9
  testSig_HLSDem_PWinPosLoCurr_mp : Outport  Port=10
  testSig_HLSDem_PWinNegLoCurr_mp : Outport  Port=11
  testSig_HLSDem_KiLoCurr_mp : Outport  Port=12
  testSig_HLSDem_KiPosLoCurr_mp : Outport  Port=13
  testSig_HLSDem_KiNegLoCurr_mp : Outport  Port=14
  testSig_HLSDem_IWinPosLoCurr_mp : Outport  Port=15
  testSig_HLSDem_IWinNegLoCurr_mp : Outport  Port=16
  testSig_HLSDem_KpHiCurr_mp : Outport  Port=17
  testSig_HLSDem_KpPosHiCurr_mp : Outport  Port=18
  testSig_HLSDem_KpNegHiCurr_mp : Outport  Port=19
  testSig_HLSDem_PWinPosHiCurr_mp : Outport  Port=20
  testSig_HLSDem_PWinNegHiCurr_mp : Outport  Port=21
  testSig_HLSDem_KiHiCurr_mp : Outport  Port=22
  testSig_HLSDem_KiPosHiCurr_mp : Outport  Port=23
  testSig_HLSDem_KiNegHiCurr_mp : Outport  Port=24
  testSig_HLSDem_IWinPosHiCurr_mp : Outport  Port=25
  testSig_HLSDem_IWinNegHiCurr_mp : Outport  Port=26
  testSig_DrvDem_nSetPLo : Outport  Port=27
  testSig_DrvDem_nSetPHi : Outport  Port=28
  testSig_DrvDem_KpCurrLo_mp : Outport  Port=29
  testSig_DrvDem_KpPosCurrLo_mp : Outport  Port=30
  testSig_DrvDem_KpNegCurrLo_mp : Outport  Port=31
  testSig_DrvDem_PWinPosLo : Outport  Port=32
  testSig_DrvDem_PWinNegLo : Outport  Port=33
  testSig_DrvDem_KiCurrLo_mp : Outport  Port=34
  testSig_DrvDem_KiPosCurrLo_mp : Outport  Port=35
  testSig_DrvDem_KiNegCurrLo_mp : Outport  Port=36
  testSig_DrvDem_IWinPosLo : Outport  Port=37
  testSig_DrvDem_IWinNegLo : Outport  Port=38
  testSig_DrvDem_KpCurrHi_mp : Outport  Port=39
  testSig_DrvDem_KpPosCurrHi_mp : Outport  Port=40
  testSig_DrvDem_KpNegCurrHi_mp : Outport  Port=41
  testSig_DrvDem_PWinPosHi : Outport  Port=42
  testSig_DrvDem_PWinNegHi : Outport  Port=43
  testSig_DrvDem_KiCurrHi_mp : Outport  Port=44
  testSig_DrvDem_KiPosCurrHi_mp : Outport  Port=45
  testSig_DrvDem_KiNegCurrHi_mp : Outport  Port=46
  testSig_DrvDem_IWinPosHi : Outport  Port=47
  testSig_DrvDem_IWinNegHi : Outport  Port=48
  testSig_HLSDem_trqReq : Outport  Port=49
  testSig_DrvDem_trqReq : Outport  Port=50
  testSig_WESDem_KpCurrHi_mp : Outport  Port=51
  testSig_WESDem_KpCurrLo_mp : Outport  Port=52
  testSig_WESDem_KpPosCurrHi_mp : Outport  Port=53
  testSig_WESDem_KpPosCurrLo_mp : Outport  Port=54
  testSig_WESDem_KpNegCurrHi_mp : Outport  Port=55
  testSig_WESDem_KpNegCurrLo_mp : Outport  Port=56
  testSig_WESDem_PWinPosHi : Outport  Port=57
  testSig_WESDem_PWinPosLo : Outport  Port=58
  testSig_WESDem_PWinNegHi : Outport  Port=59
  testSig_WESDem_PWinNegLo : Outport  Port=60
  testSig_WESDem_KiCurrHi_mp : Outport  Port=61
  testSig_WESDem_KiCurrLo_mp : Outport  Port=62
  testSig_WESDem_KiNegCurrHi_mp : Outport  Port=63
  testSig_WESDem_KiNegCurrLo_mp : Outport  Port=64
  testSig_WESDem_KiPosCurrHi_mp : Outport  Port=65
  testSig_WESDem_KiPosCurrLo_mp : Outport  Port=66
  testSig_WESDem_IWinNegHi : Outport  Port=67
  testSig_WESDem_IWinNegLo : Outport  Port=68
  testSig_WESDem_IWinPosHi : Outport  Port=69
  testSig_WESDem_IWinPosLo : Outport  Port=70
  testSig_WESDem_trqReq : Outport  Port=71
  testSig_WESDem_nSetPHi : Outport  Port=72
  testSig_WESDem_nSetPLo : Outport  Port=73
  testSig_ExtDem_KpCurrHi_mp : Outport  Port=74
  testSig_ExtDem_KpCurrLo_mp : Outport  Port=75
  testSig_ExtDem_KpNegCurrHi_mp : Outport  Port=76
  testSig_ExtDem_KpNegCurrLo_mp : Outport  Port=77
  testSig_ExtDem_KpPosCurrHi_mp : Outport  Port=78
  testSig_ExtDem_KpPosCurrLo_mp : Outport  Port=79
  testSig_ExtDem_PWinPosHi : Outport  Port=80
  testSig_ExtDem_PWinPosLo : Outport  Port=81
  testSig_ExtDem_PWinNegHi : Outport  Port=82
  testSig_ExtDem_PWinNegLo : Outport  Port=83
  testSig_ExtDem_KiCurrHi_mp : Outport  Port=84
  testSig_ExtDem_KiCurrLo_mp : Outport  Port=85
  testSig_ExtDem_KiNegCurrHi_mp : Outport  Port=86
  testSig_ExtDem_KiNegCurrLo_mp : Outport  Port=87
  testSig_ExtDem_KiPosCurrHi_mp : Outport  Port=88
  testSig_ExtDem_KiPosCurrLo_mp : Outport  Port=89
  testSig_ExtDem_IWinPosHi : Outport  Port=90
  testSig_ExtDem_IWinPosLo : Outport  Port=91
  testSig_ExtDem_IWinNegHi : Outport  Port=92
  testSig_ExtDem_IWinNegLo : Outport  Port=93
  testSig_ExtDem_nSetPHi : Outport  Port=94
  testSig_ExtDem_nSetPLo : Outport  Port=95
  testSig_ExtDem_trqReq : Outport  Port=96
  testSig_Epm_nEng : Outport  Port=97
  testSig_T15_st : Outport  Port=98
  sig_Req_Bus : Outport  Port=99
  wires:
  BS/1 -> testSig_EISGov_st1/1  "<testSig_EISGov_st1>"
  BS/2 -> testSig_EISGov_st3/1  "<testSig_EISGov_st3>"
  BS/3 -> testSig_EISGov_st6/1  "<testSig_EISGov_st6>"
  BS/4 -> testSig_EISGov_st7/1  "<testSig_EISGov_st7>"
  BS/5 -> testSig_HLSDem_nSetPLo/1  "<testSig_HLSDem_nSetPLo>"
  BS/6 -> testSig_HLSDem_nSetPHi/1  "<testSig_HLSDem_nSetPHi>"
  BS/7 -> testSig_HLSDem_KpLoCurr_mp/1  "<testSig_HLSDem_KpLoCurr_mp>"
  BS/8 -> testSig_HLSDem_KpPosLoCurr_mp/1  "<testSig_HLSDem_KpPosLoCurr_mp>"
  BS/9 -> testSig_HLSDem_KpNegLoCurr_mp/1  "<testSig_HLSDem_KpNegLoCurr_mp>"
  BS/10 -> testSig_HLSDem_PWinPosLoCurr_mp/1  "<testSig_HLSDem_PWinPosLoCurr_mp>"
  BS/11 -> testSig_HLSDem_PWinNegLoCurr_mp/1  "<testSig_HLSDem_PWinNegLoCurr_mp>"
  BS/12 -> testSig_HLSDem_KiLoCurr_mp/1  "<testSig_HLSDem_KiLoCurr_mp>"
  BS/13 -> testSig_HLSDem_KiPosLoCurr_mp/1  "<testSig_HLSDem_KiPosLoCurr_mp>"
  BS/14 -> testSig_HLSDem_KiNegLoCurr_mp/1  "<testSig_HLSDem_KiNegLoCurr_mp>"
  BS/15 -> testSig_HLSDem_IWinPosLoCurr_mp/1  "<testSig_HLSDem_IWinPosLoCurr_mp>"
  BS/16 -> testSig_HLSDem_IWinNegLoCurr_mp/1  "<testSig_HLSDem_IWinNegLoCurr_mp>"
  BS/17 -> testSig_HLSDem_KpHiCurr_mp/1  "<testSig_HLSDem_KpHiCurr_mp>"
  BS/18 -> testSig_HLSDem_KpPosHiCurr_mp/1  "<testSig_HLSDem_KpPosHiCurr_mp>"
  BS/19 -> testSig_HLSDem_KpNegHiCurr_mp/1  "<testSig_HLSDem_KpNegHiCurr_mp>"
  BS/20 -> testSig_HLSDem_PWinPosHiCurr_mp/1  "<testSig_HLSDem_PWinPosHiCurr_mp>"
  BS/21 -> testSig_HLSDem_PWinNegHiCurr_mp/1  "<testSig_HLSDem_PWinNegHiCurr_mp>"
  BS/22 -> testSig_HLSDem_KiHiCurr_mp/1  "<testSig_HLSDem_KiHiCurr_mp>"
  BS/23 -> testSig_HLSDem_KiPosHiCurr_mp/1  "<testSig_HLSDem_KiPosHiCurr_mp>"
  BS/24 -> testSig_HLSDem_KiNegHiCurr_mp/1  "<testSig_HLSDem_KiNegHiCurr_mp>"
  BS/25 -> testSig_HLSDem_IWinPosHiCurr_mp/1  "<testSig_HLSDem_IWinPosHiCurr_mp>"
  BS/26 -> testSig_HLSDem_IWinNegHiCurr_mp/1  "<testSig_HLSDem_IWinNegHiCurr_mp>"
  BS/27 -> testSig_DrvDem_nSetPLo/1  "<testSig_DrvDem_nSetPLo>"
  BS/28 -> testSig_DrvDem_nSetPHi/1  "<testSig_DrvDem_nSetPHi>"
  BS/29 -> testSig_DrvDem_KpCurrLo_mp/1  "<testSig_DrvDem_KpCurrLo_mp>"
  BS/30 -> testSig_DrvDem_KpPosCurrLo_mp/1  "<testSig_DrvDem_KpPosCurrLo_mp>"
  BS/31 -> testSig_DrvDem_KpNegCurrLo_mp/1  "<testSig_DrvDem_KpNegCurrLo_mp>"
  BS/32 -> testSig_DrvDem_PWinPosLo/1  "<testSig_DrvDem_PWinPosLo>"
  BS/33 -> testSig_DrvDem_PWinNegLo/1  "<testSig_DrvDem_PWinNegLo>"
  BS/34 -> testSig_DrvDem_KiCurrLo_mp/1  "<testSig_DrvDem_KiCurrLo_mp>"
  BS/35 -> testSig_DrvDem_KiPosCurrLo_mp/1  "<testSig_DrvDem_KiPosCurrLo_mp>"
  BS/36 -> testSig_DrvDem_KiNegCurrLo_mp/1  "<testSig_DrvDem_KiNegCurrLo_mp>"
  BS/37 -> testSig_DrvDem_IWinPosLo/1  "<testSig_DrvDem_IWinPosLo>"
  BS/38 -> testSig_DrvDem_IWinNegLo/1  "<testSig_DrvDem_IWinNegLo>"
  BS/39 -> testSig_DrvDem_KpCurrHi_mp/1  "<testSig_DrvDem_KpCurrHi_mp>"
  BS/40 -> testSig_DrvDem_KpPosCurrHi_mp/1  "<testSig_DrvDem_KpPosCurrHi_mp>"
  BS/41 -> testSig_DrvDem_KpNegCurrHi_mp/1  "<testSig_DrvDem_KpNegCurrHi_mp>"
  BS/42 -> testSig_DrvDem_PWinPosHi/1  "<testSig_DrvDem_PWinPosHi>"
  BS/43 -> testSig_DrvDem_PWinNegHi/1  "<testSig_DrvDem_PWinNegHi>"
  BS/44 -> testSig_DrvDem_KiCurrHi_mp/1  "<testSig_DrvDem_KiCurrHi_mp>"
  BS/45 -> testSig_DrvDem_KiPosCurrHi_mp/1  "<testSig_DrvDem_KiPosCurrHi_mp>"
  BS/46 -> testSig_DrvDem_KiNegCurrHi_mp/1  "<testSig_DrvDem_KiNegCurrHi_mp>"
  BS/47 -> testSig_DrvDem_IWinPosHi/1  "<testSig_DrvDem_IWinPosHi>"
  BS/48 -> testSig_DrvDem_IWinNegHi/1  "<testSig_DrvDem_IWinNegHi>"
  BS/49 -> testSig_HLSDem_trqReq/1  "<testSig_HLSDem_trqReq>"
  BS/50 -> testSig_DrvDem_trqReq/1  "<testSig_DrvDem_trqReq>"
  BS/51 -> testSig_WESDem_KpCurrHi_mp/1  "<testSig_WESDem_KpCurrHi_mp>"
  BS/52 -> testSig_WESDem_KpCurrLo_mp/1  "<testSig_WESDem_KpCurrLo_mp>"
  BS/53 -> testSig_WESDem_KpPosCurrHi_mp/1  "<testSig_WESDem_KpPosCurrHi_mp>"
  BS/54 -> testSig_WESDem_KpPosCurrLo_mp/1  "<testSig_WESDem_KpPosCurrLo_mp>"
  BS/55 -> testSig_WESDem_KpNegCurrHi_mp/1  "<testSig_WESDem_KpNegCurrHi_mp>"
  BS/56 -> testSig_WESDem_KpNegCurrLo_mp/1  "<testSig_WESDem_KpNegCurrLo_mp>"
  BS/57 -> testSig_WESDem_PWinPosHi/1  "<testSig_WESDem_PWinPosHi>"
  BS/58 -> testSig_WESDem_PWinPosLo/1  "<testSig_WESDem_PWinPosLo>"
  BS/59 -> testSig_WESDem_PWinNegHi/1  "<testSig_WESDem_PWinNegHi>"
  BS/60 -> testSig_WESDem_PWinNegLo/1  "<testSig_WESDem_PWinNegLo>"
  BS/61 -> testSig_WESDem_KiCurrHi_mp/1  "<testSig_WESDem_KiCurrHi_mp>"
  BS/62 -> testSig_WESDem_KiCurrLo_mp/1  "<testSig_WESDem_KiCurrLo_mp>"
  BS/63 -> testSig_WESDem_KiNegCurrHi_mp/1  "<testSig_WESDem_KiNegCurrHi_mp>"
  BS/64 -> testSig_WESDem_KiNegCurrLo_mp/1  "<testSig_WESDem_KiNegCurrLo_mp>"
  BS/65 -> testSig_WESDem_KiPosCurrHi_mp/1  "<testSig_WESDem_KiPosCurrHi_mp>"
  BS/66 -> testSig_WESDem_KiPosCurrLo_mp/1  "<testSig_WESDem_KiPosCurrLo_mp>"
  BS/67 -> testSig_WESDem_IWinNegHi/1  "<testSig_WESDem_IWinNegHi>"
  BS/68 -> testSig_WESDem_IWinNegLo/1  "<testSig_WESDem_IWinNegLo>"
  BS/69 -> testSig_WESDem_IWinPosHi/1  "<testSig_WESDem_IWinPosHi>"
  BS/70 -> testSig_WESDem_IWinPosLo/1  "<testSig_WESDem_IWinPosLo>"
  BS/71 -> testSig_WESDem_trqReq/1  "<testSig_WESDem_trqReq>"
  BS/72 -> testSig_WESDem_nSetPHi/1  "<testSig_WESDem_nSetPHi>"
  BS/73 -> testSig_WESDem_nSetPLo/1  "<testSig_WESDem_nSetPLo>"
  BS/74 -> testSig_ExtDem_KpCurrHi_mp/1  "<testSig_ExtDem_KpCurrHi_mp>"
  BS/75 -> testSig_ExtDem_KpCurrLo_mp/1  "<testSig_ExtDem_KpCurrLo_mp>"
  BS/76 -> testSig_ExtDem_KpNegCurrHi_mp/1  "<testSig_ExtDem_KpNegCurrHi_mp>"
  BS/77 -> testSig_ExtDem_KpNegCurrLo_mp/1  "<testSig_ExtDem_KpNegCurrLo_mp>"
  BS/78 -> testSig_ExtDem_KpPosCurrHi_mp/1  "<testSig_ExtDem_KpPosCurrHi_mp>"
  BS/79 -> testSig_ExtDem_KpPosCurrLo_mp/1  "<testSig_ExtDem_KpPosCurrLo_mp>"
  BS/80 -> testSig_ExtDem_PWinPosHi/1  "<testSig_ExtDem_PWinPosHi>"
  BS/81 -> testSig_ExtDem_PWinPosLo/1  "<testSig_ExtDem_PWinPosLo>"
  BS/82 -> testSig_ExtDem_PWinNegHi/1  "<testSig_ExtDem_PWinNegHi>"
  BS/83 -> testSig_ExtDem_PWinNegLo/1  "<testSig_ExtDem_PWinNegLo>"
  BS/84 -> testSig_ExtDem_KiCurrHi_mp/1  "<testSig_ExtDem_KiCurrHi_mp>"
  BS/85 -> testSig_ExtDem_KiCurrLo_mp/1  "<testSig_ExtDem_KiCurrLo_mp>"
  BS/86 -> testSig_ExtDem_KiNegCurrHi_mp/1  "<testSig_ExtDem_KiNegCurrHi_mp>"
  BS/87 -> testSig_ExtDem_KiNegCurrLo_mp/1  "<testSig_ExtDem_KiNegCurrLo_mp>"
  BS/88 -> testSig_ExtDem_KiPosCurrHi_mp/1  "<testSig_ExtDem_KiPosCurrHi_mp>"
  BS/89 -> testSig_ExtDem_KiPosCurrLo_mp/1  "<testSig_ExtDem_KiPosCurrLo_mp>"
  BS/90 -> testSig_ExtDem_IWinPosHi/1  "<testSig_ExtDem_IWinPosHi>"
  BS/91 -> testSig_ExtDem_IWinPosLo/1  "<testSig_ExtDem_IWinPosLo>"
  BS/92 -> testSig_ExtDem_IWinNegHi/1  "<testSig_ExtDem_IWinNegHi>"
  BS/93 -> testSig_ExtDem_IWinNegLo/1  "<testSig_ExtDem_IWinNegLo>"
  BS/94 -> testSig_ExtDem_nSetPHi/1  "<testSig_ExtDem_nSetPHi>"
  BS/95 -> testSig_ExtDem_nSetPLo/1  "<testSig_ExtDem_nSetPLo>"
  BS/96 -> testSig_ExtDem_trqReq/1  "<testSig_ExtDem_trqReq>"
  BS/97 -> testSig_Epm_nEng/1  "<testSig_Epm_nEng>"
  BS/98 -> testSig_T15_st/1  "<testSig_T15_st>"
  testSignals_R001/1(testSignals) -> BS/1, sig_Req_Bus/1

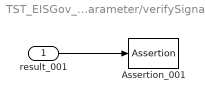
== system TST_EISGov_SelectParameter/verifySignals ==
  result_001 : Inport
  Assertion_001 : Assertion  Enabled=off
  wires:
  result_001/1 -> Assertion_001/1
